simulink model "q2"  (R2023a)
settings: Solver=VariableStepAuto  StartTime=0.0  StopTime=10.0  RelTol=1e-3
libraries: simulink x1
settings Model: Creator=giri0  LastModifiedBy=giri0

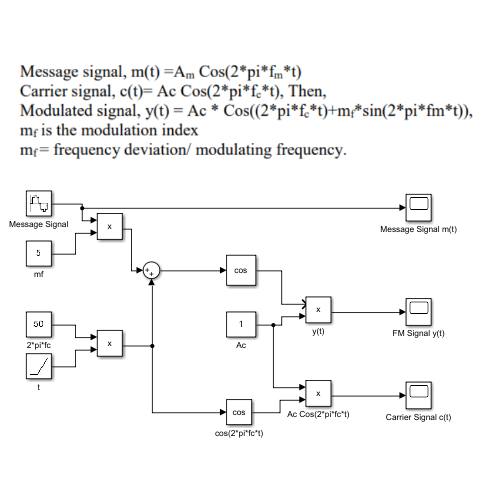
[thumbnail: Simulink's stored preview of the top-level diagram]
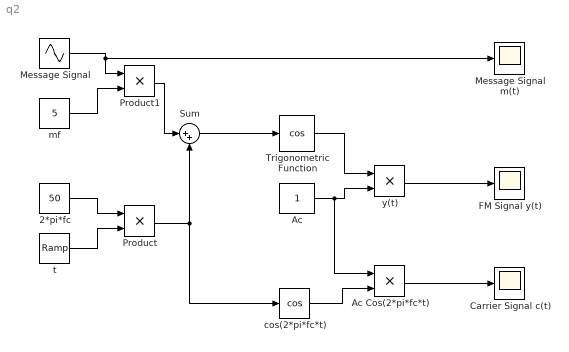
== system q2 ==
  2*pi*fc : Constant  Value=50
  Ac : Constant
  Ac Cos(2*pi*fc*t) : Product
  Carrier Signal c(t) : Scope
  FM Signal y(t) : Scope
  Message Signal : Sin  Frequency=2*pi  SampleTime=1/5000
  Message Signal m(t) : Scope
  Product : Product
  Product1 : Product
  Sum : Sum  Inputs=|++
  Trigonometric Function : Trigonometry  Operator=cos
  cos(2*pi*fc*t) : Trigonometry  Operator=cos
  mf : Constant  Value=5
  t : simulink/Sources/Ramp  slope=1  start=0  InitialOutput=0
  y(t) : Product
  wires:
  t/1 -> Product/2
  2*pi*fc/1 -> Product/1
  Product/1 -> cos(2*pi*fc*t)/1, Sum/2
  Product1/1 -> Sum/1
  mf/1 -> Product1/2
  Message Signal/1 -> Message Signal m(t)/1, Product1/1
  Sum/1 -> Trigonometric Function/1
  Ac/1 -> Ac Cos(2*pi*fc*t)/1, y(t)/2
  Trigonometric Function/1 -> y(t)/1
  y(t)/1 -> FM Signal y(t)/1
  cos(2*pi*fc*t)/1 -> Ac Cos(2*pi*fc*t)/2
  Ac Cos(2*pi*fc*t)/1 -> Carrier Signal c(t)/1
